simulink model "ownStateSpaceModel"  (R2015a)
settings: Solver=ode4  StartTime=0.0  StopTime=2  RelTol=1e-3
values from neighbouring files (symbols this model uses):
  A = A - B*k'    [example1.m]    (also in example2.m = [-0.00819, -25.70839, 0, -32.17095; - 0.00019, -1.27626, 1, ; example3.m = [-0.00819, -25.70839, 0, -32.17095; - 0.00019, -1.27626, 1, ; rscale.m = a; rscale2.m = a)
  B = [0; 4]    [example1.m]    (also in example2.m = [-6.80939;-0.14968;-14.06111;0]; example3.m = [-6.80939, 0;-0.14968, 0;-14.06111, 0;0, 0]; rscale.m = b; rscale2.m = b)
  C = eye(2)    [example1.m]    (also in example2.m = [0 1 0 0]; example3.m = [0 1 0 0; 0 1 0 0]; rscale.m = c; rscale2.m = c)
  D = [0; 0]    [example1.m]    (also in example2.m = [0]; example3.m = [0 0; 0 0]; rscale.m = d; rscale2.m = d)
  k = [8.09; 16.5]    [example1.m]
  x0 = [1.0;0]    [example1.m]
settings Model: Creator=adamfelis  LastModifiedBy=Qba

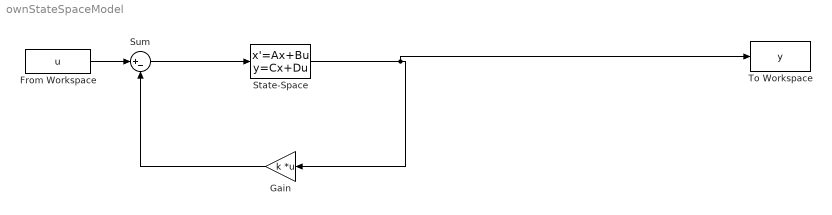
== system ownStateSpaceModel ==
  From Workspace : FromWorkspace  VariableName=u  SampleTime=0
  Gain : Gain  Gain=k  Multiplication=Matrix(K*u)
  State-Space : StateSpace  A=A  B=B  C=C  D=D  X0=x0
  Sum : Sum  Inputs=|+-
  To Workspace : ToWorkspace  VariableName=y  SaveFormat=Timeseries  SampleTime=-1
  wires:
  State-Space/1 -> To Workspace/1, Gain/1
  From Workspace/1 -> Sum/1
  Sum/1 -> State-Space/1
  Gain/1 -> Sum/2
